simulink model "Converters"  (R2024b)
settings: Solver=VariableStepAuto  StartTime=0.0  StopTime=10.0  RelTol=1e-3
settings Model: Creator=Ahmad  LastModifiedBy=Ahmad

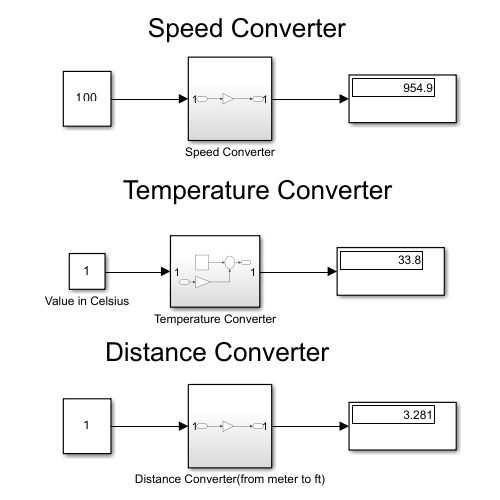
[thumbnail: Simulink's stored preview of the top-level diagram]
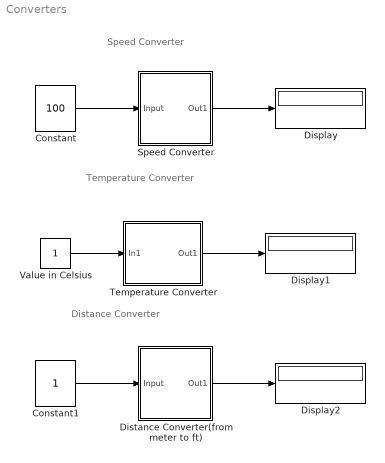
== system Converters ==
  note: Temperature Converter
  note: Speed Converter
  note: Distance Converter
  Constant : Constant  Value=100
  Constant1 : Constant
  Display : Display
  Display1 : Display
  Display2 : Display
  Distance Converter(from meter to ft) : Subsystem
  Speed Converter : Subsystem
  Temperature Converter : Subsystem
  Value in Celsius : Constant
  wires:
  Constant/1 -> Speed Converter/1(Input)
  Speed Converter/1(Out1) -> Display/1
  Value in Celsius/1 -> Temperature Converter/1(In1)
  Temperature Converter/1(Out1) -> Display1/1
  Constant1/1 -> Distance Converter(from meter to ft)/1(Input)
  Distance Converter(from meter to ft)/1(Out1) -> Display2/1

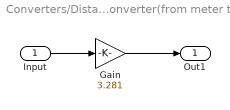
== system Converters/Distance Converter(from meter to ft) ==
  Input : Inport
  Gain : Gain  Gain=3.281
  Out1 : Outport
  wires:
  Input/1 -> Gain/1
  Gain/1 -> Out1/1

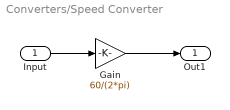
== system Converters/Speed Converter ==
  Input : Inport
  Gain : Gain  Gain=60/(2*pi)
  Out1 : Outport
  wires:
  Input/1 -> Gain/1
  Gain/1 -> Out1/1

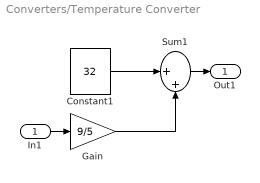
== system Converters/Temperature Converter ==
  In1 : Inport
  Constant1 : Constant  Value=32
  Gain : Gain  Gain=9/5
  Sum1 : Sum  Inputs=|++
  Out1 : Outport
  wires:
  Constant1/1 -> Sum1/1
  Sum1/1 -> Out1/1
  Gain/1 -> Sum1/2
  In1/1 -> Gain/1
